simulink model "body_simulink"  (R2016a)
settings: Solver=VariableStepAuto  StartTime=0.0  StopTime=40.0  RelTol=1e-3
libraries: dspsrcs4 x1, simulink_extras x1
settings Model: Creator=patty  LastModifiedBy=patty

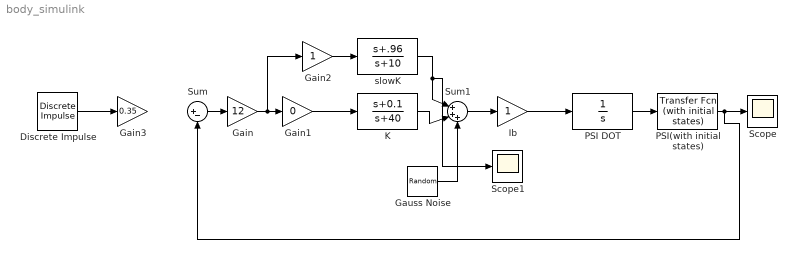
== system body_simulink ==
  Discrete Impulse : dspsrcs4/Discrete  Impulse  Delay=0  SampleTime=1  FrameSample=1  OutputFrames=off  dataType=double  isSigned=on  wordLen=16  udDataType=sfix(16)  fracBitsMode=Best precision  numFracBits=15  OutDataTypeStr=double  LastOutDataTypeStr=double
  Gain : Gain  Gain=12
  Gain1 : Gain  Gain=0
  Gain2 : Gain
  Gain3 : Gain  Gain=0.35
  Gauss Noise : RandomNumber  Variance=0.05  SampleTime=0.1
  Ib : Gain
  K : TransferFcn  Numerator=[1 0.1]  Denominator=[1 40]
  PSI DOT : TransferFcn  Denominator=[1 0]
  PSI(with initial states) : simulink_extras/Additional Linear/Transfer Fcn (with initial states)  N=[1]  D=[1 0]  X0=.35
  Scope : Scope
  Scope1 : Scope
  Sum : Sum  Inputs=|+-
  Sum1 : Sum  Inputs=|+++
  slowK : TransferFcn  Numerator=[1 .96]  Denominator=[1 10]
  wires:
  Discrete Impulse/1 -> Gain3/1
  PSI(with initial states)/1 -> Sum/2, Scope/1
  PSI DOT/1 -> PSI(with initial states)/1
  Sum1/1 -> Ib/1
  Sum/1 -> Gain/1
  Gain/1 -> Gain2/1, Gain1/1
  Gauss Noise/1 -> Sum1/3
  K/1 -> Sum1/2
  slowK/1 -> Scope1/1, Sum1/1
  Gain1/1 -> K/1
  Gain2/1 -> slowK/1
  Ib/1 -> PSI DOT/1
